simulink model "system"  (R2024b)
settings: Solver=FixedStepDiscrete  StartTime=0.0  StopTime=10.0  RelTol=1e-3
model workspace (MAT data in the model file):
  Risks = Simulink.Bus
  Risks.Alignment = -1
  Risks.PreserveElementDimensions = 0
  Risks.Elements_internal(1) = Simulink.BusElement
  Risks.Elements_internal(1).DimensionsMode = 'Fixed'
  Risks.Elements_internal(1).SamplingMode = 'Sample based'
  Risks.Elements_internal(1).SampleTime = -1
  Risks.Elements_internal(1).Name = 'VaR'
  Risks.Elements_internal(1).DataType_internal = 'double'
  Risks.Elements_internal(1).Complexity = 'real'
  Risks.Elements_internal(1).Dimensions = 1
  Risks.Elements_internal(2) = Simulink.BusElement
  Risks.Elements_internal(2).DimensionsMode = 'Fixed'
  Risks.Elements_internal(2).SamplingMode = 'Sample based'
  Risks.Elements_internal(2).SampleTime = -1
  Risks.Elements_internal(2).Name = 'liquidity'
  Risks.Elements_internal(2).DataType_internal = 'double'
  Risks.Elements_internal(2).Complexity = 'real'
  Risks.Elements_internal(2).Dimensions = 1
  Risks.Elements_internal(3) = Simulink.BusElement
  Risks.Elements_internal(3).DimensionsMode = 'Fixed'
  Risks.Elements_internal(3).SamplingMode = 'Sample based'
  Risks.Elements_internal(3).SampleTime = -1
  Risks.Elements_internal(3).Name = 'correlation'
  Risks.Elements_internal(3).DataType_internal = 'double'
  Risks.Elements_internal(3).Complexity = 'real'
  Risks.Elements_internal(3).Dimensions = 1
  Risks.Elements_internal(4) = Simulink.BusElement
  Risks.Elements_internal(4).DimensionsMode = 'Fixed'
  Risks.Elements_internal(4).SamplingMode = 'Sample based'
  Risks.Elements_internal(4).SampleTime = -1
  Risks.Elements_internal(4).Name = 'wavelet_coherence'
  Risks.Elements_internal(4).DataType_internal = 'double'
  Risks.Elements_internal(4).Complexity = 'real'
  Risks.Elements_internal(4).Dimensions = 1
  Risks.Elements_internal(5) = Simulink.BusElement
  Risks.Elements_internal(5).DimensionsMode = 'Fixed'
  Risks.Elements_internal(5).SamplingMode = 'Sample based'
  Risks.Elements_internal(5).SampleTime = -1
  Risks.Elements_internal(5).Name = 'crossMFDFA'
  Risks.Elements_internal(5).DataType_internal = 'double'
  Risks.Elements_internal(5).Complexity = 'real'
  Risks.Elements_internal(5).Dimensions = 1
  Risks.DataScope = 'Auto'
undefined symbols (not defined in the file): AA, Risk, UI
settings Model: Creator=lenskiy  LastModifiedBy=nagi
settings OptimizationCC: EnhancedBackFolding=on  PassReuseOutputArgsThreshold=0  ZeroExternalMemoryAtStartup=off  ZeroInternalMemoryAtStartup=off  MaxStackSize=64  OptimizeBlockOrder=speed  DifferentSizesBufferReuse=on  OptimizationCustomize=off
settings DebuggingCC: ParameterTunabilityLossMsg=error
settings HardwareCC: ProdBitPerLong=64  ProdHWDeviceType=Intel->x86-64 (MAC OS X)  UseEmbeddedCoderFeatures=off
settings SFSimCC: MATLABDynamicMemAlloc=off
settings RTWCC: Description=Embedded Coder  SystemTargetFile=ert.tlc  HardwareBoard=Robot Operating System 2 (ROS 2)  TLCOptions="-aInlineSetEventsForThisBaseRateFcn=TLC_FALSE -aSuppressMultiTaskScheduler=TLC_FALSE  -aRateBasedStepFcn=0"  TemplateMakefile=ert_default_tmf  Toolchain=Colcon Tools  TargetLang=C++
settings CodeAppCC: ForceParamTrailComments=on  OperatorAnnotations=on
settings ERTTargetCC: ERTCustomFileBanners=off  CodeInterfacePackaging=C++ class  SupportContinuousTime=on  SupportNonInlinedSFcns=on  RemoveResetFunc=off  ModelStepFunctionPrototypeControlCompliant=off  InlinedParameterPlacement=Hierarchical  RootIOFormat=Structure reference  DynamicArrayContainerType=coder::array

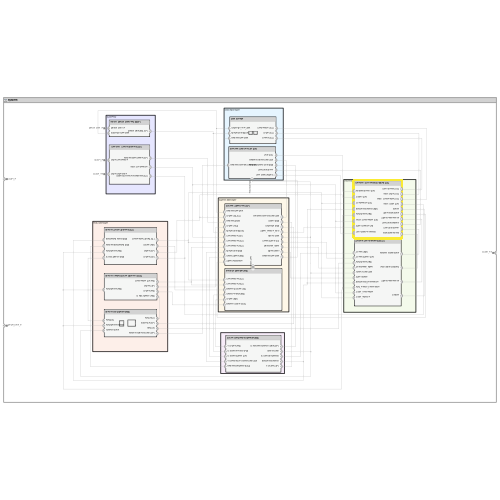
[thumbnail: Simulink's stored preview of the top-level diagram]
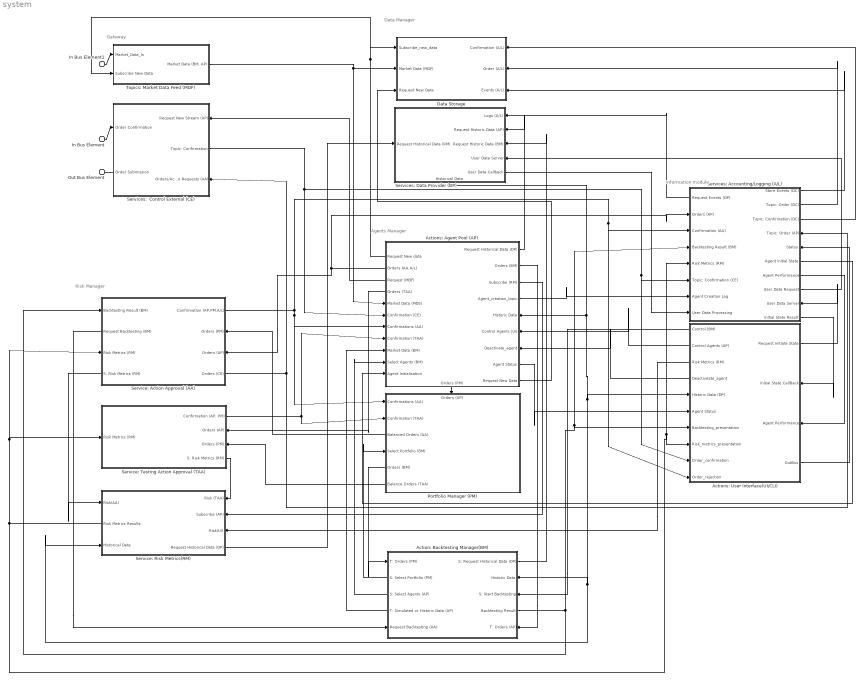
== system system ==
  note: Agents Manager
  note: Risk Manager
  note: Information module
  note: Data Manager
  note: Gateway
  In Bus Element : Inport  PortName=CCAPI_in
  In Bus Element1 : Inport  Port=2  PortName=Market_Data_In
  "  Services:  Control External (CE)" : Subsystem
      settings: PortSchema="{\"entries\":[{\"content\":{\"headerSize\":26,\"margin\":15,\"minimumSpacing\":25,\"sides\":[{\"content\":{\"connectorIds\":[\"In3\",\"Out1\"]},\"type\":\"ConnectorPlacement.EquallySpacedRectSide\",\"uuid\":\"c7e54eda-a439-456a-891f-e8c098e73b96\"},{\"content\":{\"connectorIds\":[\"In1\",\"Out2\",\"In2\"],\"side\":\"RIGHT\"},\"type\":\"ConnectorPlacement.EquallySpacedRectSide\",\"uuid\":\"93d01d87-f209-49b1-9fea-6a6e1e49cb0b\"},{\"content\":{\"side\":\"TOP\"},\"type\":\"ConnectorPlacement.EquallySpacedRectSide\",\"uuid\":\"f0abbd0b-06c8-4244-9bda-d971a55bccc5\"},{\"content\":{\"side\":\"BOTTOM\"},\"type\":\"ConnectorPlacement.EquallySpacedRectSide\",\"uuid\":\"d0091bd5-d57f-475a-8bc6-bc66948a1d1d\"}]},\"type\":\"ConnectorPlacement.EquallySpacedConnector\",\"uuid\":\"cf42f307-3a29-44ef-94e0-20f9bb6c1c81\"}],\"packageUris\":[\"http://schema.mathworks.com/mf0/Connector/R2020b\"],\"version\":\"1.0\"}"
  "Action: Backtesting Manager(BM) " : Subsystem
      settings: PortSchema="{\"entries\":[{\"content\":{\"headerSize\":26,\"margin\":15,\"minimumSpacing\":25,\"sides\":[{\"content\":{\"connectorIds\":[\"In4\",\"Out2\",\"Out4\",\"Out3\",\"In3\"]},\"type\":\"ConnectorPlacement.EquallySpacedRectSide\",\"uuid\":\"c7e54eda-a439-456a-891f-e8c098e73b96\"},{\"content\":{\"connectorIds\":[\"Out5\",\"In1\",\"In2\",\"Out1\",\"In5\"],\"side\":\"RIGHT\"},\"type\":\"ConnectorPlacement.EquallySpacedRectSide\",\"uuid\":\"93d01d87-f209-49b1-9fea-6a6e1e49cb0b\"},{\"content\":{\"side\":\"TOP\"},\"type\":\"ConnectorPlacement.EquallySpacedRectSide\",\"uuid\":\"f0abbd0b-06c8-4244-9bda-d971a55bccc5\"},{\"content\":{\"side\":\"BOTTOM\"},\"type\":\"ConnectorPlacement.EquallySpacedRectSide\",\"uuid\":\"c7ce6db1-31da-416d-9401-48a4b61b54ad\"}]},\"type\":\"ConnectorPlacement.EquallySpacedConnector\",\"uuid\":\"cf42f307-3a29-44ef-94e0-20f9bb6c1c81\"}],\"packageUris\":[\"http://schema.mathworks.com/mf0/Connector/R2020b\"],\"version\":\"1.0\"}"
  Actions: Agent Pool (AP) : Subsystem
      settings: PortSchema="{\"entries\":[{\"content\":{\"headerSize\":26,\"margin\":15,\"minimumSpacing\":25,\"sides\":[{\"content\":{\"connectorIds\":[\"Out8\",\"Out6\",\"Out5\",\"Out2\",\"In8\",\"In4\",\"In7\",\"In3\",\"In6\",\"In2\",\"In10\"]},\"type\":\"ConnectorPlacement.EquallySpacedRectSide\",\"uuid\":\"c7e54eda-a439-456a-891f-e8c098e73b96\"},{\"content\":{\"connectorIds\":[\"Out7\",\"Out3\",\"Out4\",\"Out10\",\"In1\",\"In5\",\"In9\",\"Out9\",\"Out11\"],\"side\":\"RIGHT\"},\"type\":\"ConnectorPlacement.EquallySpacedRectSide\",\"uuid\":\"93d01d87-f209-49b1-9fea-6a6e1e49cb0b\"},{\"content\":{\"side\":\"TOP\"},\"type\":\"ConnectorPlacement.EquallySpacedRectSide\",\"uuid\":\"f0abbd0b-06c8-4244-9bda-d971a55bccc5\"},{\"content\":{\"connectorIds\":[\"Out1\"],\"side\":\"BOTTOM\"},\"type\":\"ConnectorPlacement.EquallySpacedRectSide\",\"uuid\":\"897f63fa-91c4-4177-8500-44381925c77f\"}]},\"type\":\"ConnectorPlacement.EquallySpacedConnector\",\"uuid\":\"cf42f307-3a29-44ef-94e0-20f9bb6c1c81\"}],\"packageUris\":[\"http://schema.mathworks.com/mf0/Connector/R2020b\"],\"version\":\"1.0\"}"
  Actions: User Interface(UI/CLI) : Subsystem
      settings: PortSchema="{\"entries\":[{\"content\":{\"headerSize\":26,\"margin\":15,\"minimumSpacing\":25,\"sides\":[{\"content\":{\"connectorIds\":[\"Out3\",\"Out4\",\"Out2\",\"Out6\",\"In1\",\"In3\",\"In4\",\"In5\",\"In6\",\"In7\"]},\"type\":\"ConnectorPlacement.EquallySpacedRectSide\",\"uuid\":\"c7e54eda-a439-456a-891f-e8c098e73b96\"},{\"content\":{\"connectorIds\":[\"Out5\",\"In2\",\"In8\",\"Out1\"],\"side\":\"RIGHT\"},\"type\":\"ConnectorPlacement.EquallySpacedRectSide\",\"uuid\":\"93d01d87-f209-49b1-9fea-6a6e1e49cb0b\"},{\"content\":{\"side\":\"TOP\"},\"type\":\"ConnectorPlacement.EquallySpacedRectSide\",\"uuid\":\"f0abbd0b-06c8-4244-9bda-d971a55bccc5\"},{\"content\":{\"side\":\"BOTTOM\"},\"type\":\"ConnectorPlacement.EquallySpacedRectSide\",\"uuid\":\"239dc4b0-7955-4c14-b3b1-3030c8a0e9ad\"}]},\"type\":\"ConnectorPlacement.EquallySpacedConnector\",\"uuid\":\"cf42f307-3a29-44ef-94e0-20f9bb6c1c81\"}],\"packageUris\":[\"http://schema.mathworks.com/mf0/Connector/R2020b\"],\"version\":\"1.0\"}"
  Data Storage : Subsystem
      settings: PortSchema="{\"entries\":[{\"content\":{\"headerSize\":26,\"margin\":15,\"minimumSpacing\":25,\"sides\":[{\"content\":{\"connectorIds\":[\"In5\",\"In2\",\"In6\"]},\"type\":\"ConnectorPlacement.EquallySpacedRectSide\",\"uuid\":\"c7e54eda-a439-456a-891f-e8c098e73b96\"},{\"content\":{\"connectorIds\":[\"In3\",\"In4\",\"In1\"],\"side\":\"RIGHT\"},\"type\":\"ConnectorPlacement.EquallySpacedRectSide\",\"uuid\":\"93d01d87-f209-49b1-9fea-6a6e1e49cb0b\"},{\"content\":{\"side\":\"TOP\"},\"type\":\"ConnectorPlacement.EquallySpacedRectSide\",\"uuid\":\"f0abbd0b-06c8-4244-9bda-d971a55bccc5\"},{\"content\":{\"side\":\"BOTTOM\"},\"type\":\"ConnectorPlacement.EquallySpacedRectSide\",\"uuid\":\"d3fd7ded-18bf-4804-97b5-79887e5eea75\"}]},\"type\":\"ConnectorPlacement.EquallySpacedConnector\",\"uuid\":\"cf42f307-3a29-44ef-94e0-20f9bb6c1c81\"}],\"packageUris\":[\"http://schema.mathworks.com/mf0/Connector/R2020b\"],\"version\":\"1.0\"}"
  Portfolio Manager (PM) : Subsystem
      settings: PortSchema="{\"entries\":[{\"content\":{\"headerSize\":26,\"margin\":15,\"minimumSpacing\":25,\"sides\":[{\"content\":{\"connectorIds\":[\"In2\",\"In4\",\"Out3\",\"In1\",\"Out1\",\"Out2\"]},\"type\":\"ConnectorPlacement.EquallySpacedRectSide\",\"uuid\":\"c7e54eda-a439-456a-891f-e8c098e73b96\"},{\"content\":{\"side\":\"RIGHT\"},\"type\":\"ConnectorPlacement.EquallySpacedRectSide\",\"uuid\":\"93d01d87-f209-49b1-9fea-6a6e1e49cb0b\"},{\"content\":{\"connectorIds\":[\"In3\"],\"side\":\"TOP\"},\"type\":\"ConnectorPlacement.EquallySpacedRectSide\",\"uuid\":\"f0abbd0b-06c8-4244-9bda-d971a55bccc5\"},{\"content\":{\"side\":\"BOTTOM\"},\"type\":\"ConnectorPlacement.EquallySpacedRectSide\",\"uuid\":\"c17b4fb6-208b-4b15-8ab9-f7677697b6e9\"}]},\"type\":\"ConnectorPlacement.EquallySpacedConnector\",\"uuid\":\"cf42f307-3a29-44ef-94e0-20f9bb6c1c81\"}],\"packageUris\":[\"http://schema.mathworks.com/mf0/Connector/R2020b\"],\"version\":\"1.0\"}"
  Service: Action Approval (AA) : Subsystem
      settings: PortSchema="{\"entries\":[{\"content\":{\"headerSize\":26,\"margin\":15,\"minimumSpacing\":25,\"sides\":[{\"content\":{\"connectorIds\":[\"In1\",\"Out4\",\"In4\",\"Out1\"]},\"type\":\"ConnectorPlacement.EquallySpacedRectSide\",\"uuid\":\"c7e54eda-a439-456a-891f-e8c098e73b96\"},{\"content\":{\"connectorIds\":[\"Out3\",\"In2\",\"In3\",\"Out2\"],\"side\":\"RIGHT\"},\"type\":\"ConnectorPlacement.EquallySpacedRectSide\",\"uuid\":\"93d01d87-f209-49b1-9fea-6a6e1e49cb0b\"},{\"content\":{\"side\":\"TOP\"},\"type\":\"ConnectorPlacement.EquallySpacedRectSide\",\"uuid\":\"f0abbd0b-06c8-4244-9bda-d971a55bccc5\"},{\"content\":{\"side\":\"BOTTOM\"},\"type\":\"ConnectorPlacement.EquallySpacedRectSide\",\"uuid\":\"404a1439-590f-4a61-8168-47d1c9a050f4\"}]},\"type\":\"ConnectorPlacement.EquallySpacedConnector\",\"uuid\":\"cf42f307-3a29-44ef-94e0-20f9bb6c1c81\"}],\"packageUris\":[\"http://schema.mathworks.com/mf0/Connector/R2020b\"],\"version\":\"1.0\"}"
  Service: Risk Metrics(RM) : Subsystem
      settings: PortSchema="{\"entries\":[{\"content\":{\"headerSize\":26,\"margin\":15,\"minimumSpacing\":25,\"sides\":[{\"content\":{\"connectorIds\":[\"In3\",\"Out1\",\"In5\"]},\"type\":\"ConnectorPlacement.EquallySpacedRectSide\",\"uuid\":\"c7e54eda-a439-456a-891f-e8c098e73b96\"},{\"content\":{\"connectorIds\":[\"In1\",\"In4\",\"In2\",\"Out2\"],\"side\":\"RIGHT\"},\"type\":\"ConnectorPlacement.EquallySpacedRectSide\",\"uuid\":\"93d01d87-f209-49b1-9fea-6a6e1e49cb0b\"},{\"content\":{\"side\":\"TOP\"},\"type\":\"ConnectorPlacement.EquallySpacedRectSide\",\"uuid\":\"f0abbd0b-06c8-4244-9bda-d971a55bccc5\"},{\"content\":{\"side\":\"BOTTOM\"},\"type\":\"ConnectorPlacement.EquallySpacedRectSide\",\"uuid\":\"1a2f452a-f007-439c-b229-615c9b87871c\"}]},\"type\":\"ConnectorPlacement.EquallySpacedConnector\",\"uuid\":\"cf42f307-3a29-44ef-94e0-20f9bb6c1c81\"}],\"packageUris\":[\"http://schema.mathworks.com/mf0/Connector/R2020b\"],\"version\":\"1.0\"}"
  Service: Testing Action Approval (TAA) : Subsystem
      settings: PortSchema="{\"entries\":[{\"content\":{\"headerSize\":26,\"margin\":15,\"minimumSpacing\":25,\"sides\":[{\"content\":{\"connectorIds\":[\"In3\"]},\"type\":\"ConnectorPlacement.EquallySpacedRectSide\",\"uuid\":\"c7e54eda-a439-456a-891f-e8c098e73b96\"},{\"content\":{\"connectorIds\":[\"Out2\",\"In2\",\"In1\",\"Out1\"],\"side\":\"RIGHT\"},\"type\":\"ConnectorPlacement.EquallySpacedRectSide\",\"uuid\":\"93d01d87-f209-49b1-9fea-6a6e1e49cb0b\"},{\"content\":{\"side\":\"TOP\"},\"type\":\"ConnectorPlacement.EquallySpacedRectSide\",\"uuid\":\"f0abbd0b-06c8-4244-9bda-d971a55bccc5\"},{\"content\":{\"side\":\"BOTTOM\"},\"type\":\"ConnectorPlacement.EquallySpacedRectSide\",\"uuid\":\"404a1439-590f-4a61-8168-47d1c9a050f4\"}]},\"type\":\"ConnectorPlacement.EquallySpacedConnector\",\"uuid\":\"cf42f307-3a29-44ef-94e0-20f9bb6c1c81\"}],\"packageUris\":[\"http://schema.mathworks.com/mf0/Connector/R2020b\"],\"version\":\"1.0\"}"
  Services: Accounting/Logging (A/L) : Subsystem
      settings: PortSchema="{\"entries\":[{\"content\":{\"headerSize\":26,\"margin\":15,\"minimumSpacing\":25,\"sides\":[{\"content\":{\"connectorIds\":[\"Out1\",\"In1\",\"In2\",\"In6\",\"In7\",\"In4\",\"In8\",\"In9\"]},\"type\":\"ConnectorPlacement.EquallySpacedRectSide\",\"uuid\":\"c7e54eda-a439-456a-891f-e8c098e73b96\"},{\"content\":{\"connectorIds\":[\"Out2\",\"Out4\",\"Out3\",\"In5\",\"In3\",\"Out5\",\"Out6\",\"Out7\",\"In10\",\"Out8\"],\"side\":\"RIGHT\"},\"type\":\"ConnectorPlacement.EquallySpacedRectSide\",\"uuid\":\"93d01d87-f209-49b1-9fea-6a6e1e49cb0b\"},{\"content\":{\"side\":\"TOP\"},\"type\":\"ConnectorPlacement.EquallySpacedRectSide\",\"uuid\":\"f0abbd0b-06c8-4244-9bda-d971a55bccc5\"},{\"content\":{\"side\":\"BOTTOM\"},\"type\":\"ConnectorPlacement.EquallySpacedRectSide\",\"uuid\":\"8932d7e1-f270-4d28-9443-134a4dd6acae\"}]},\"type\":\"ConnectorPlacement.EquallySpacedConnector\",\"uuid\":\"cf42f307-3a29-44ef-94e0-20f9bb6c1c81\"}],\"packageUris\":[\"http://schema.mathworks.com/mf0/Connector/R2020b\"],\"version\":\"1.0\"}"
  Services: Data Provider (DP) : Subsystem
      settings: PortSchema="{\"entries\":[{\"content\":{\"headerSize\":26,\"margin\":15,\"minimumSpacing\":25,\"sides\":[{\"content\":{\"connectorIds\":[\"In4\"]},\"type\":\"ConnectorPlacement.EquallySpacedRectSide\",\"uuid\":\"c7e54eda-a439-456a-891f-e8c098e73b96\"},{\"content\":{\"connectorIds\":[\"In1\",\"In3\",\"In2\",\"In5\",\"Out2\"],\"side\":\"RIGHT\"},\"type\":\"ConnectorPlacement.EquallySpacedRectSide\",\"uuid\":\"93d01d87-f209-49b1-9fea-6a6e1e49cb0b\"},{\"content\":{\"side\":\"TOP\"},\"type\":\"ConnectorPlacement.EquallySpacedRectSide\",\"uuid\":\"f0abbd0b-06c8-4244-9bda-d971a55bccc5\"},{\"content\":{\"connectorIds\":[\"Out1\"],\"side\":\"BOTTOM\"},\"type\":\"ConnectorPlacement.EquallySpacedRectSide\",\"uuid\":\"d3fd7ded-18bf-4804-97b5-79887e5eea75\"}]},\"type\":\"ConnectorPlacement.EquallySpacedConnector\",\"uuid\":\"cf42f307-3a29-44ef-94e0-20f9bb6c1c81\"}],\"packageUris\":[\"http://schema.mathworks.com/mf0/Connector/R2020b\"],\"version\":\"1.0\"}"
  Topics: Market Data Feed (MDF) : Subsystem
      settings: PortSchema="{\"entries\":[{\"content\":{\"headerSize\":26,\"margin\":15,\"minimumSpacing\":25,\"sides\":[{\"content\":{\"connectorIds\":[\"In1\",\"In2\"]},\"type\":\"ConnectorPlacement.EquallySpacedRectSide\",\"uuid\":\"c7e54eda-a439-456a-891f-e8c098e73b96\"},{\"content\":{\"connectorIds\":[\"Out1\"],\"side\":\"RIGHT\"},\"type\":\"ConnectorPlacement.EquallySpacedRectSide\",\"uuid\":\"93d01d87-f209-49b1-9fea-6a6e1e49cb0b\"},{\"content\":{\"side\":\"TOP\"},\"type\":\"ConnectorPlacement.EquallySpacedRectSide\",\"uuid\":\"f0abbd0b-06c8-4244-9bda-d971a55bccc5\"},{\"content\":{\"side\":\"BOTTOM\"},\"type\":\"ConnectorPlacement.EquallySpacedRectSide\",\"uuid\":\"d0091bd5-d57f-475a-8bc6-bc66948a1d1d\"}]},\"type\":\"ConnectorPlacement.EquallySpacedConnector\",\"uuid\":\"cf42f307-3a29-44ef-94e0-20f9bb6c1c81\"}],\"packageUris\":[\"http://schema.mathworks.com/mf0/Connector/R2020b\"],\"version\":\"1.0\"}"
  Out Bus Element : Outport  PortName=CCAPI_out
  wires:
  Topics: Market Data Feed (MDF)/1("Market Data (BM, AP)") -> Actions: Agent Pool (AP)/8(Market Data (MDS)), Data Storage/2(Market Data (MDF))
  Actions: Agent Pool (AP)/6(Orders (AA,A/L)) -> Service: Action Approval (AA)/3(Orders (AP)), Services: Accounting/Logging (A/L)/1(Orders (AP))
  Service: Action Approval (AA)/3(Confirmation (AP,PM,A/L)) -> Actions: User Interface(UI/CLI)/7(Order_rejection), Services: Accounting/Logging (A/L)/2(Confirmation (AA)), Portfolio Manager (PM)/2(Confirmations (AA)), Actions: Agent Pool (AP)/7(Confirmations (AA))
  Service: Action Approval (AA)/2(Orders (CE)) -> "  Services:  Control External (CE)"/2(Orders/Account Info Requests (AA)), Services: Accounting/Logging (A/L)/5(Topic: Order (AP))
  Service: Action Approval (AA)/1(S: Risk Metrics (RM)) -> Service: Risk Metrics(RM)/3(Risk(AA))
  Services: Data Provider (DP)/1(Historical Data) -> Service: Risk Metrics(RM)/5(Historical Data), "Action: Backtesting Manager(BM) "/1(Historic Data), Actions: User Interface(UI/CLI)/1(Historic Data (DP)), Actions: Agent Pool (AP)/1(Historic Data)
  Actions: User Interface(UI/CLI)/1(OutBus) -> Services: Accounting/Logging (A/L)/3(" Status")
  Actions: Agent Pool (AP)/5(Request (MDF)) -> "  Services:  Control External (CE)"/1(Request New Stream (AP))
  "Action: Backtesting Manager(BM) "/5(S: Request Historical Data (DP)) -> Services: Data Provider (DP)/2(Request Historic Data (BM))
  Services: Accounting/Logging (A/L)/2(Store Events (DC)) -> Data Storage/1(" Events (A/L)")
  "Action: Backtesting Manager(BM) "/4(S: Select Agents (AP)) -> Actions: Agent Pool (AP)/2(Select Agents (BM))
  "Action: Backtesting Manager(BM) "/3(T: Simulated or Historic Data (AP)) -> Actions: Agent Pool (AP)/6(Market Data (BM))
  Actions: Agent Pool (AP)/3(Orders (BM)) -> "Action: Backtesting Manager(BM) "/5(T: Orders (AP))
  Actions: User Interface(UI/CLI)/4(Control Agents (AP)) -> Actions: Agent Pool (AP)/5(Control Agents (UI))
  Actions: User Interface(UI/CLI)/3(Control (BM)) -> "Action: Backtesting Manager(BM) "/2(S: Start Backtesting)
  Actions: User Interface(UI/CLI)/2(Risk Metrics (RM)) -> Service: Risk Metrics(RM)/2(Risk(UI))
  Actions: Agent Pool (AP)/1(Orders (PM)) -> Portfolio Manager (PM)/3(Orders (AP))
  Portfolio Manager (PM)/3(Balanced Orders (AA)) -> Service: Action Approval (AA)/2(Orders (PM))
  Portfolio Manager (PM)/1(Orders (BM)) -> "Action: Backtesting Manager(BM) "/4(T: Orders (PM))
  "Action: Backtesting Manager(BM) "/2(S: Select Portfolio (PM)) -> Portfolio Manager (PM)/1(Select Portfolio (BM))
  Services: Accounting/Logging (A/L)/1(Request Events (DP)) -> Services: Data Provider (DP)/1(" Logs (A/L)")
  Actions: Agent Pool (AP)/2(Orders (TAA)) -> Service: Testing Action Approval (TAA)/2(Orders (AP))
  Service: Testing Action Approval (TAA)/2("Confirmation (AP, PM)") -> Actions: Agent Pool (AP)/3(Confirmation (TAA)), Portfolio Manager (PM)/4(Confirmation (TAA))
  Portfolio Manager (PM)/2(Balance Orders (TAA)) -> Service: Testing Action Approval (TAA)/1(Orders (PM))
  Service: Testing Action Approval (TAA)/1(S: Risk Metrics (RM)) -> Service: Risk Metrics(RM)/1(Risk (TAA))
  Service: Risk Metrics(RM)/1(Risk Metrics Results) -> Service: Action Approval (AA)/4(Risk Metrics (RM)), Service: Testing Action Approval (TAA)/3(Risk Metrics (RM)), Services: Accounting/Logging (A/L)/7(Risk Metrics (RM)), Actions: User Interface(UI/CLI)/5(Risk_metrics_presentation)
  Actions: Agent Pool (AP)/4(Subscribe (RM)) -> Service: Risk Metrics(RM)/4(Subscribe (AP))
  "  Services:  Control External (CE)"/1(Order Submission) -> Out Bus Element/1
  In Bus Element/1 -> "  Services:  Control External (CE)"/3(Order Confirmation)
  "  Services:  Control External (CE)"/2(Topic: Confirmation) -> Actions: Agent Pool (AP)/4(Confirmation (CE)), Actions: User Interface(UI/CLI)/6(Order_confirmation), Services: Accounting/Logging (A/L)/4(Topic: Confirmation (CE))
  Services: Accounting/Logging (A/L)/3(Topic: Confirmation (DC)) -> Data Storage/3(Confirmation (A/L))
  Services: Accounting/Logging (A/L)/4(Topic: Order (DC)) -> Data Storage/4(Order (A/L))
  In Bus Element1/1 -> Topics: Market Data Feed (MDF)/1(Market_Data_In)
  Service: Action Approval (AA)/4(Request Backtesting (BM)) -> "Action: Backtesting Manager(BM) "/3(Request Backtesting (AA))
  "Action: Backtesting Manager(BM) "/1(Backtesting Result) -> Services: Accounting/Logging (A/L)/6(Backtesting Result (BM)), Actions: User Interface(UI/CLI)/4(Backtesting_presentation), Service: Action Approval (AA)/1(Backtesting Result (BM))
  Actions: Agent Pool (AP)/7(Request Historical Data (DP)) -> Services: Data Provider (DP)/3(Request Historic Data (AP))
  Service: Risk Metrics(RM)/2(Request Historical Data (DP)) -> Services: Data Provider (DP)/4(Request Historical Data (RM))
  Actions: Agent Pool (AP)/8(Request New data) -> Topics: Market Data Feed (MDF)/2(Subscribe New Data), Data Storage/5(Subscribe_new_data)
  Services: Data Provider (DP)/2(User Data Callback) -> Services: Accounting/Logging (A/L)/9(User Data Processing)
  Actions: Agent Pool (AP)/9(Agent Status) -> Actions: User Interface(UI/CLI)/3(Agent Status)
  Actions: Agent Pool (AP)/10(Agent_creation_topic) -> Services: Accounting/Logging (A/L)/8(Agent Creation Log)
  Actions: User Interface(UI/CLI)/6(Deactiveate_agent) -> Actions: Agent Pool (AP)/9(Deactivate_agent)
  Actions: Agent Pool (AP)/11(Request New Data) -> Data Storage/6(Request New Data)
  Services: Accounting/Logging (A/L)/5(Agent Initial State) -> Actions: Agent Pool (AP)/10(Agent Initialisation)
  Services: Accounting/Logging (A/L)/6(Agent Performance) -> Actions: User Interface(UI/CLI)/8(Agent Performance)
  Services: Accounting/Logging (A/L)/7(User Data Request) -> Services: Data Provider (DP)/5(User Data Server)
  Actions: User Interface(UI/CLI)/5(Request Initiate State) -> Services: Accounting/Logging (A/L)/10(User Data Server)
  Services: Accounting/Logging (A/L)/8(Initial State Result) -> Actions: User Interface(UI/CLI)/2(Initial State CallBack)

== system system/  Services:  Control External (CE) ==
  Bus Element In2 : Inport  PortName=Request New Stream (AP)
  Bus Element In1 : Inport  Port=2  PortName=Orders/Account Info Requests (AA)
  Bus Element In3 : Inport  Port=3  PortName=Order Confirmation
  Bus Element Out3 : Outport  PortName=Order Submission
  Bus Element Out4 : Outport  Port=2  PortName=Topic: Confirmation

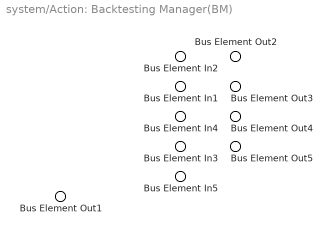
== system system/Action: Backtesting Manager(BM)  ==
  Bus Element In5 : Inport  PortName=Historic Data
  Bus Element In1 : Inport  Port=2  PortName=S: Start Backtesting
  Bus Element In3 : Inport  Port=3  PortName=Request Backtesting (AA)
  Bus Element In2 : Inport  Port=4  PortName=T: Orders (PM)
  Bus Element In4 : Inport  Port=5  PortName=T: Orders (AP)
  Bus Element Out4 : Outport  PortName=Backtesting Result
  Bus Element Out5 : Outport  Port=2  PortName=S: Select Portfolio (PM)
  Bus Element Out3 : Outport  Port=3  PortName=T: Simulated or Historic Data (AP)
  Bus Element Out2 : Outport  Port=4  PortName=S: Select Agents (AP)
  Bus Element Out1 : Outport  Port=5  PortName=S: Request Historical Data (DP)

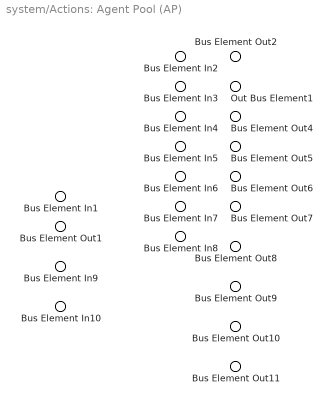
== system system/Actions: Agent Pool (AP) ==
  Bus Element In7 : Inport  PortName=Historic Data
  Bus Element In2 : Inport  Port=2  PortName=Select Agents (BM)
  Bus Element In6 : Inport  Port=3  PortName=Confirmation (TAA)
  Bus Element In8 : Inport  Port=4  PortName=Confirmation (CE)
  Bus Element In4 : Inport  Port=5  PortName=Control Agents (UI)
  Bus Element In5 : Inport  Port=6  PortName=Market Data (BM)
  Bus Element In3 : Inport  Port=7  PortName=Confirmations (AA)
  Bus Element In1 : Inport  Port=8  PortName=Market Data (MDS)
  Bus Element In9 : Inport  Port=9  PortName=Deactivate_agent
  Bus Element In10 : Inport  Port=10  PortName=Agent Initialisation
  Bus Element Out5 : Outport  PortName=Orders (PM)
  Bus Element Out6 : Outport  Port=2  PortName=Orders (TAA)
  Bus Element Out4 : Outport  Port=3  PortName=Orders (BM)
  Bus Element Out7 : Outport  Port=4  PortName=Subscribe (RM)
  Bus Element Out2 : Outport  Port=5  PortName=Request (MDF)
  Bus Element Out1 : Outport  Port=6  PortName=Orders (AA,A/L)
  Out Bus Element1 : Outport  Port=7  PortName=Request Historical Data (DP)
  Bus Element Out8 : Outport  Port=8  PortName=Request New data
  Bus Element Out9 : Outport  Port=9  PortName=Agent Status
  Bus Element Out10 : Outport  Port=10  PortName=Agent_creation_topic
  Bus Element Out11 : Outport  Port=11  PortName=Request New Data

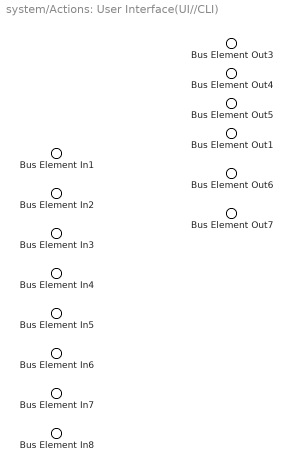
== system system/Actions: User Interface(UI//CLI) ==
  Bus Element In1 : Inport  PortName=Historic Data (DP)
  Bus Element In2 : Inport  Port=2  PortName=Initial State CallBack
  Bus Element In3 : Inport  Port=3  PortName=Agent Status
  Bus Element In4 : Inport  Port=4  PortName=Backtesting_presentation
  Bus Element In5 : Inport  Port=5  PortName=Risk_metrics_presentation
  Bus Element In6 : Inport  Port=6  PortName=Order_confirmation
  Bus Element In7 : Inport  Port=7  PortName=Order_rejection
  Bus Element In8 : Inport  Port=8  PortName=Agent Performance
  Bus Element Out1 : Outport  PortName=OutBus
  Bus Element Out5 : Outport  Port=2  PortName=Risk Metrics (RM)
  Bus Element Out4 : Outport  Port=3  PortName=Control (BM)
  Bus Element Out3 : Outport  Port=4  PortName=Control Agents (AP)
  Bus Element Out6 : Outport  Port=5  PortName=Request Initiate State
  Bus Element Out7 : Outport  Port=6  PortName=Deactiveate_agent

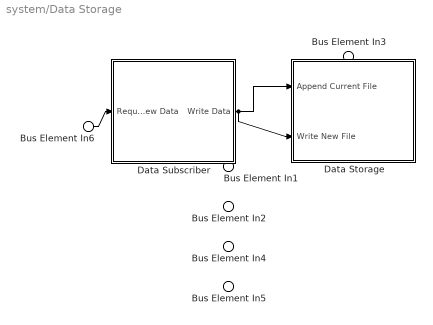
== system system/Data Storage ==
  Bus Element In3 : Inport  PortName=Events (A/L)
  Bus Element In1 : Inport  Port=2  PortName=Market Data (MDF)
  Bus Element In2 : Inport  Port=3  PortName=Confirmation (A/L)
  Bus Element In4 : Inport  Port=4  PortName=Order (A/L)
  Bus Element In5 : Inport  Port=5  PortName=Subscribe_new_data
  Bus Element In6 : Inport  Port=6  PortName=Request New Data
  Data Storage : Subsystem
      settings: PortSchema="{\"entries\":[{\"content\":{\"headerSize\":26,\"margin\":15,\"minimumSpacing\":25,\"sides\":[{\"content\":{\"connectorIds\":[\"In1\",\"In2\"]},\"type\":\"ConnectorPlacement.EquallySpacedRectSide\",\"uuid\":\"72b088da-6be2-4f39-86d9-1dec5d939a57\"},{\"content\":{\"side\":\"RIGHT\"},\"type\":\"ConnectorPlacement.EquallySpacedRectSide\",\"uuid\":\"3e630222-beed-4269-8eaa-e743757a473d\"},{\"content\":{\"side\":\"TOP\"},\"type\":\"ConnectorPlacement.EquallySpacedRectSide\",\"uuid\":\"e55fff88-3bcb-47c6-8712-517af8558fc3\"}]},\"type\":\"ConnectorPlacement.EquallySpacedConnector\",\"uuid\":\"d9b8126a-9f7a-4470-914d-1cf46528a28d\"}],\"packageUris\":[\"http://schema.mathworks.com/mf0/Connector/R2020b\"],\"version\":\"1.0\"}"
  Data Subscriber : Subsystem
      settings: PortSchema="{\"entries\":[{\"content\":{\"headerSize\":26,\"margin\":15,\"minimumSpacing\":25,\"sides\":[{\"content\":{\"connectorIds\":[\"In1\"]},\"type\":\"ConnectorPlacement.EquallySpacedRectSide\",\"uuid\":\"72b088da-6be2-4f39-86d9-1dec5d939a57\"},{\"content\":{\"connectorIds\":[\"Out1\"],\"side\":\"RIGHT\"},\"type\":\"ConnectorPlacement.EquallySpacedRectSide\",\"uuid\":\"3e630222-beed-4269-8eaa-e743757a473d\"},{\"content\":{\"side\":\"TOP\"},\"type\":\"ConnectorPlacement.EquallySpacedRectSide\",\"uuid\":\"e55fff88-3bcb-47c6-8712-517af8558fc3\"}]},\"type\":\"ConnectorPlacement.EquallySpacedConnector\",\"uuid\":\"d9b8126a-9f7a-4470-914d-1cf46528a28d\"}],\"packageUris\":[\"http://schema.mathworks.com/mf0/Connector/R2020b\"],\"version\":\"1.0\"}"
  wires:
  Data Subscriber/1(Write Data) -> Data Storage/2(Write New File), Data Storage/1(Append Current File)
  Bus Element In6/1 -> Data Subscriber/1(Request New Data)

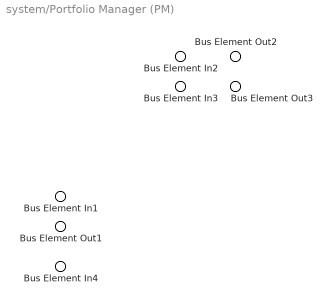
== system system/Portfolio Manager (PM) ==
  Bus Element In3 : Inport  PortName=Select Portfolio (BM)
  Bus Element In2 : Inport  Port=2  PortName=Confirmations (AA)
  Bus Element In1 : Inport  Port=3  PortName=Orders (AP)
  Bus Element In4 : Inport  Port=4  PortName=Confirmation (TAA)
  Bus Element Out2 : Outport  PortName=Orders (BM)
  Bus Element Out3 : Outport  Port=2  PortName=Balance Orders (TAA)
  Bus Element Out1 : Outport  Port=3  PortName=Balanced Orders (AA)

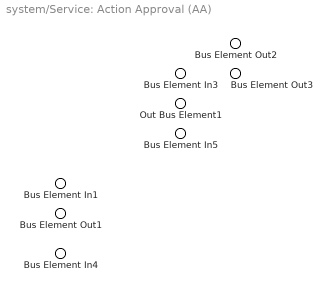
== system system/Service: Action Approval (AA) ==
  Bus Element In5 : Inport  PortName=Backtesting Result (BM)
  Bus Element In3 : Inport  Port=2  PortName=Orders (PM)
  Bus Element In1 : Inport  Port=3  PortName=Orders (AP)
  Bus Element In4 : Inport  Port=4  PortName=Risk Metrics (RM)
  Bus Element Out3 : Outport  PortName=S: Risk Metrics (RM)
  Bus Element Out2 : Outport  Port=2  PortName=Orders (CE)
  Bus Element Out1 : Outport  Port=3  PortName=Confirmation (AP,PM,A/L)
  Out Bus Element1 : Outport  Port=4  PortName=Request Backtesting (BM)

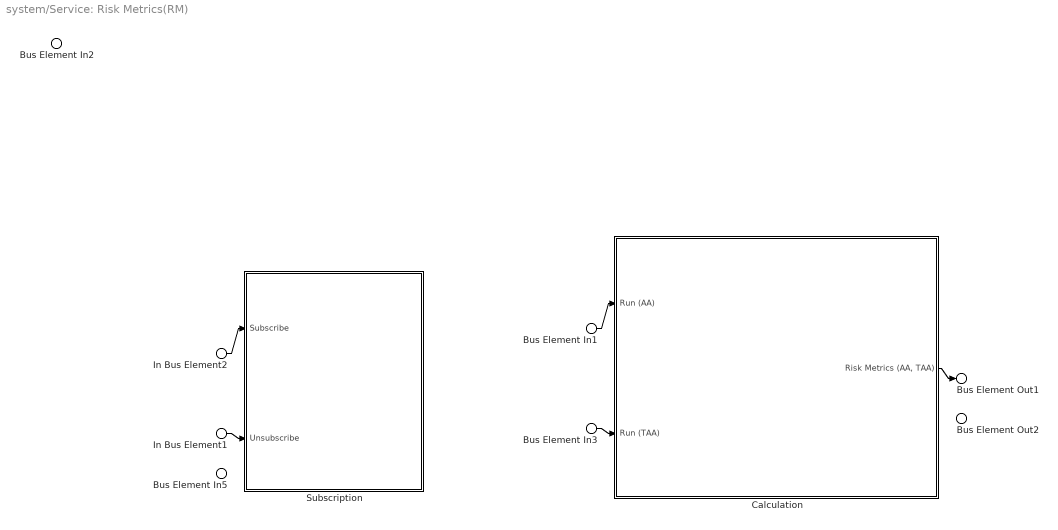
== system system/Service: Risk Metrics(RM) ==
  Bus Element In3 : Inport  PortName=Risk (TAA)
  Bus Element In2 : Inport  Port=2  PortName=Risk(UI)
  Bus Element In1 : Inport  Port=3  PortName=Risk(AA)
  In Bus Element2 : Inport  Port=4  PortName=Subscribe (AP)
  In Bus Element1 : Inport  Port=4  PortName=Subscribe (AP)
  Bus Element In5 : Inport  Port=5  PortName=Historical Data
  Calculation : Subsystem
      settings: PortSchema="{\"entries\":[{\"content\":{\"headerSize\":26,\"margin\":15,\"minimumSpacing\":25,\"sides\":[{\"content\":{\"connectorIds\":[\"In1\",\"In2\"]},\"type\":\"ConnectorPlacement.EquallySpacedRectSide\",\"uuid\":\"dd5ff5af-be48-4b61-a3ee-7d818d4cdc88\"},{\"content\":{\"connectorIds\":[\"Out1\"],\"side\":\"RIGHT\"},\"type\":\"ConnectorPlacement.EquallySpacedRectSide\",\"uuid\":\"02a6924d-a1b2-490b-997c-279faf232d36\"},{\"content\":{\"side\":\"TOP\"},\"type\":\"ConnectorPlacement.EquallySpacedRectSide\",\"uuid\":\"141c48b7-11a2-4087-8334-b2fd993d46dc\"}]},\"type\":\"ConnectorPlacement.EquallySpacedConnector\",\"uuid\":\"f405ae8c-72bf-4bdb-9e54-71737400ea90\"}],\"packageUris\":[\"http://schema.mathworks.com/mf0/Connector/R2020b\"],\"version\":\"1.0\"}"
  Subscription : Subsystem
      settings: PortSchema="{\"entries\":[{\"content\":{\"headerSize\":26,\"margin\":15,\"minimumSpacing\":25,\"sides\":[{\"content\":{\"connectorIds\":[\"In1\",\"In2\"]},\"type\":\"ConnectorPlacement.EquallySpacedRectSide\",\"uuid\":\"dd5ff5af-be48-4b61-a3ee-7d818d4cdc88\"},{\"content\":{\"side\":\"RIGHT\"},\"type\":\"ConnectorPlacement.EquallySpacedRectSide\",\"uuid\":\"02a6924d-a1b2-490b-997c-279faf232d36\"},{\"content\":{\"side\":\"TOP\"},\"type\":\"ConnectorPlacement.EquallySpacedRectSide\",\"uuid\":\"141c48b7-11a2-4087-8334-b2fd993d46dc\"}]},\"type\":\"ConnectorPlacement.EquallySpacedConnector\",\"uuid\":\"f405ae8c-72bf-4bdb-9e54-71737400ea90\"}],\"packageUris\":[\"http://schema.mathworks.com/mf0/Connector/R2020b\"],\"version\":\"1.0\"}"
  Bus Element Out1 : Outport  PortName=Risk Metrics Results
  Bus Element Out2 : Outport  Port=2  PortName=Request Historical Data (DP)
  wires:
  In Bus Element2/1 -> Subscription/1(Subscribe)
  In Bus Element1/1 -> Subscription/2(Unsubscribe)
  Bus Element In1/1 -> Calculation/1(Run (AA))
  Bus Element In3/1 -> Calculation/2(Run (TAA))
  Calculation/1("Risk Metrics (AA, TAA)") -> Bus Element Out1/1

== system system/Service: Testing Action Approval (TAA) ==
  Bus Element In3 : Inport  PortName=Orders (PM)
  Bus Element In1 : Inport  Port=2  PortName=Orders (AP)
  Bus Element In2 : Inport  Port=3  PortName=Risk Metrics (RM)
  Bus Element Out3 : Outport  PortName=S: Risk Metrics (RM)
  Bus Element Out1 : Outport  Port=2  PortName=Confirmation (AP, PM)

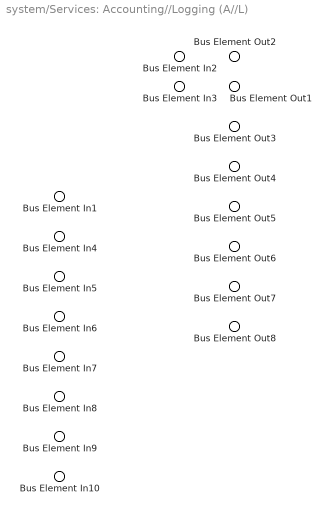
== system system/Services: Accounting//Logging (A//L) ==
  Bus Element In3 : Inport  PortName=Orders (AP)
  Bus Element In2 : Inport  Port=2  PortName=Confirmation (AA)
  Bus Element In1 : Inport  Port=3  PortName=Status
  Bus Element In4 : Inport  Port=4  PortName=Topic: Confirmation (CE)
  Bus Element In5 : Inport  Port=5  PortName=Topic: Order (AP)
  Bus Element In6 : Inport  Port=6  PortName=Backtesting Result (BM)
  Bus Element In7 : Inport  Port=7  PortName=Risk Metrics (RM)
  Bus Element In8 : Inport  Port=8  PortName=Agent Creation Log
  Bus Element In9 : Inport  Port=9  PortName=User Data Processing
  Bus Element In10 : Inport  Port=10  PortName=User Data Server
  Bus Element Out1 : Outport  PortName=Request Events (DP)
  Bus Element Out2 : Outport  Port=2  PortName=Store Events (DC)
  Bus Element Out3 : Outport  Port=3  PortName=Topic: Confirmation (DC)
  Bus Element Out4 : Outport  Port=4  PortName=Topic: Order (DC)
  Bus Element Out5 : Outport  Port=5  PortName=Agent Initial State
  Bus Element Out6 : Outport  Port=6  PortName=Agent Performance
  Bus Element Out7 : Outport  Port=7  PortName=User Data Request
  Bus Element Out8 : Outport  Port=8  PortName=Initial State Result

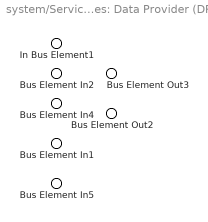
== system system/Services: Data Provider (DP) ==
  Bus Element In2 : Inport  PortName=Logs (A/L)
  Bus Element In4 : Inport  Port=2  PortName=Request Historic Data (BM)
  In Bus Element1 : Inport  Port=3  PortName=Request Historic Data (AP)
  Bus Element In1 : Inport  Port=4  PortName=Request Historical Data (RM)
  Bus Element In5 : Inport  Port=5  PortName=User Data Server
  Bus Element Out3 : Outport  PortName=Historical Data
  Bus Element Out2 : Outport  Port=2  PortName=User Data Callback

== system system/Topics: Market Data Feed (MDF) ==
  Bus Element In1 : Inport  PortName=Market_Data_In
  Bus Element In2 : Inport  Port=2  PortName=Subscribe New Data
  Bus Element Out1 : Outport  PortName=Market Data (BM, AP)

== system system/Data Storage/Data Storage ==
  Bus Element In1 : Inport  PortName=Append Current File
  Bus Element In2 : Inport  Port=2  PortName=Write New File

== system system/Data Storage/Data Subscriber ==
  Bus Element In1 : Inport  PortName=Request New Data
  Bus Element Out1 : Outport  PortName=Write Data

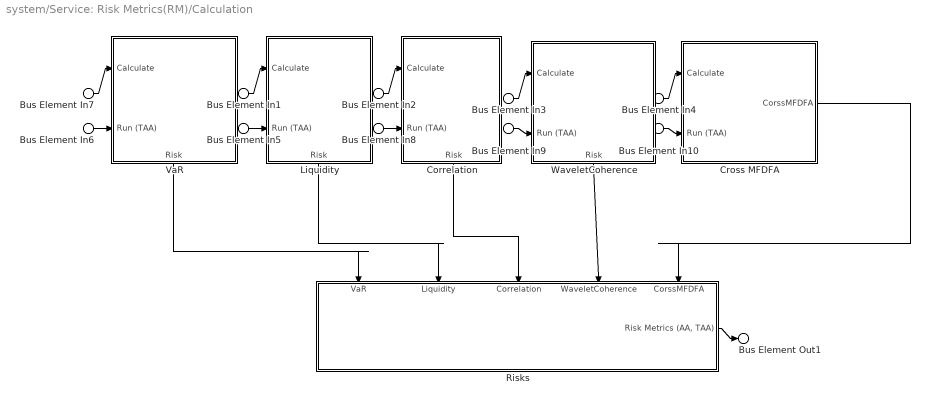
== system system/Service: Risk Metrics(RM)/Calculation ==
  Bus Element In{1..4,7} (5 alike) : Inport  PortName=Run (AA)
  Bus Element In{5..6,8..10} (5 alike) : Inport  Port=2  PortName=Run (TAA)
  Correlation : Subsystem
      settings: PortSchema="{\"entries\":[{\"content\":{\"headerSize\":26,\"margin\":15,\"minimumSpacing\":25,\"sides\":[{\"content\":{\"connectorIds\":[\"In1\",\"In2\"]},\"type\":\"ConnectorPlacement.EquallySpacedRectSide\",\"uuid\":\"dd5ff5af-be48-4b61-a3ee-7d818d4cdc88\"},{\"content\":{\"side\":\"RIGHT\"},\"type\":\"ConnectorPlacement.EquallySpacedRectSide\",\"uuid\":\"02a6924d-a1b2-490b-997c-279faf232d36\"},{\"content\":{\"side\":\"TOP\"},\"type\":\"ConnectorPlacement.EquallySpacedRectSide\",\"uuid\":\"141c48b7-11a2-4087-8334-b2fd993d46dc\"},{\"content\":{\"connectorIds\":[\"Out1\"],\"side\":\"BOTTOM\"},\"type\":\"ConnectorPlacement.EquallySpacedRectSide\",\"uuid\":\"c8d94622-5369-4926-ac8e-6b1b94c651e3\"}]},\"type\":\"ConnectorPlacement.EquallySpacedConnector\",\"uuid\":\"f405ae8c-72bf-4bdb-9e54-71737400ea90\"}],\"packageUris\":[\"http://schema.mathworks.com/mf0/Connector/R2020b\"],\"version\":\"1.0\"}"
  Cross MFDFA : Subsystem
      settings: PortSchema="{\"entries\":[{\"content\":{\"headerSize\":26,\"margin\":15,\"minimumSpacing\":25,\"sides\":[{\"content\":{\"connectorIds\":[\"In1\",\"In2\"]},\"type\":\"ConnectorPlacement.EquallySpacedRectSide\",\"uuid\":\"dd5ff5af-be48-4b61-a3ee-7d818d4cdc88\"},{\"content\":{\"connectorIds\":[\"Out1\"],\"side\":\"RIGHT\"},\"type\":\"ConnectorPlacement.EquallySpacedRectSide\",\"uuid\":\"02a6924d-a1b2-490b-997c-279faf232d36\"},{\"content\":{\"side\":\"TOP\"},\"type\":\"ConnectorPlacement.EquallySpacedRectSide\",\"uuid\":\"141c48b7-11a2-4087-8334-b2fd993d46dc\"},{\"content\":{\"side\":\"BOTTOM\"},\"type\":\"ConnectorPlacement.EquallySpacedRectSide\",\"uuid\":\"318bb783-36ea-4aa3-bd6c-38ef09b88506\"}]},\"type\":\"ConnectorPlacement.EquallySpacedConnector\",\"uuid\":\"f405ae8c-72bf-4bdb-9e54-71737400ea90\"}],\"packageUris\":[\"http://schema.mathworks.com/mf0/Connector/R2020b\"],\"version\":\"1.0\"}"
  Liquidity : Subsystem
      settings: PortSchema="{\"entries\":[{\"content\":{\"headerSize\":26,\"margin\":15,\"minimumSpacing\":25,\"sides\":[{\"content\":{\"connectorIds\":[\"In1\",\"In2\"]},\"type\":\"ConnectorPlacement.EquallySpacedRectSide\",\"uuid\":\"dd5ff5af-be48-4b61-a3ee-7d818d4cdc88\"},{\"content\":{\"side\":\"RIGHT\"},\"type\":\"ConnectorPlacement.EquallySpacedRectSide\",\"uuid\":\"02a6924d-a1b2-490b-997c-279faf232d36\"},{\"content\":{\"side\":\"TOP\"},\"type\":\"ConnectorPlacement.EquallySpacedRectSide\",\"uuid\":\"141c48b7-11a2-4087-8334-b2fd993d46dc\"},{\"content\":{\"connectorIds\":[\"Out1\"],\"side\":\"BOTTOM\"},\"type\":\"ConnectorPlacement.EquallySpacedRectSide\",\"uuid\":\"4fa86d91-e252-4fed-93db-0b64ea968a1f\"}]},\"type\":\"ConnectorPlacement.EquallySpacedConnector\",\"uuid\":\"f405ae8c-72bf-4bdb-9e54-71737400ea90\"}],\"packageUris\":[\"http://schema.mathworks.com/mf0/Connector/R2020b\"],\"version\":\"1.0\"}"
  Risks : Subsystem
      settings: PortSchema="{\"entries\":[{\"content\":{\"headerSize\":26,\"margin\":15,\"minimumSpacing\":25,\"sides\":[{\"content\":{},\"type\":\"ConnectorPlacement.EquallySpacedRectSide\",\"uuid\":\"dd5ff5af-be48-4b61-a3ee-7d818d4cdc88\"},{\"content\":{\"connectorIds\":[\"Out1\"],\"side\":\"RIGHT\"},\"type\":\"ConnectorPlacement.EquallySpacedRectSide\",\"uuid\":\"02a6924d-a1b2-490b-997c-279faf232d36\"},{\"content\":{\"connectorIds\":[\"In1\",\"In2\",\"In3\",\"In4\",\"In5\"],\"side\":\"TOP\"},\"type\":\"ConnectorPlacement.EquallySpacedRectSide\",\"uuid\":\"141c48b7-11a2-4087-8334-b2fd993d46dc\"}]},\"type\":\"ConnectorPlacement.EquallySpacedConnector\",\"uuid\":\"f405ae8c-72bf-4bdb-9e54-71737400ea90\"}],\"packageUris\":[\"http://schema.mathworks.com/mf0/Connector/R2020b\"],\"version\":\"1.0\"}"
  VaR : Subsystem
      settings: PortSchema="{\"entries\":[{\"content\":{\"headerSize\":26,\"margin\":15,\"minimumSpacing\":25,\"sides\":[{\"content\":{\"connectorIds\":[\"In1\",\"In2\"]},\"type\":\"ConnectorPlacement.EquallySpacedRectSide\",\"uuid\":\"dd5ff5af-be48-4b61-a3ee-7d818d4cdc88\"},{\"content\":{\"side\":\"RIGHT\"},\"type\":\"ConnectorPlacement.EquallySpacedRectSide\",\"uuid\":\"02a6924d-a1b2-490b-997c-279faf232d36\"},{\"content\":{\"side\":\"TOP\"},\"type\":\"ConnectorPlacement.EquallySpacedRectSide\",\"uuid\":\"141c48b7-11a2-4087-8334-b2fd993d46dc\"},{\"content\":{\"connectorIds\":[\"Out1\"],\"side\":\"BOTTOM\"},\"type\":\"ConnectorPlacement.EquallySpacedRectSide\",\"uuid\":\"b918c4be-b53c-43e3-b06e-d826fcfce314\"}]},\"type\":\"ConnectorPlacement.EquallySpacedConnector\",\"uuid\":\"f405ae8c-72bf-4bdb-9e54-71737400ea90\"}],\"packageUris\":[\"http://schema.mathworks.com/mf0/Connector/R2020b\"],\"version\":\"1.0\"}"
  WaveletCoherence : Subsystem
      settings: PortSchema="{\"entries\":[{\"content\":{\"headerSize\":26,\"margin\":15,\"minimumSpacing\":25,\"sides\":[{\"content\":{\"connectorIds\":[\"In1\",\"In2\"]},\"type\":\"ConnectorPlacement.EquallySpacedRectSide\",\"uuid\":\"dd5ff5af-be48-4b61-a3ee-7d818d4cdc88\"},{\"content\":{\"side\":\"RIGHT\"},\"type\":\"ConnectorPlacement.EquallySpacedRectSide\",\"uuid\":\"02a6924d-a1b2-490b-997c-279faf232d36\"},{\"content\":{\"side\":\"TOP\"},\"type\":\"ConnectorPlacement.EquallySpacedRectSide\",\"uuid\":\"141c48b7-11a2-4087-8334-b2fd993d46dc\"},{\"content\":{\"connectorIds\":[\"Out1\"],\"side\":\"BOTTOM\"},\"type\":\"ConnectorPlacement.EquallySpacedRectSide\",\"uuid\":\"4b4658a0-d0df-4ee1-b82c-ffc500e3ac80\"}]},\"type\":\"ConnectorPlacement.EquallySpacedConnector\",\"uuid\":\"f405ae8c-72bf-4bdb-9e54-71737400ea90\"}],\"packageUris\":[\"http://schema.mathworks.com/mf0/Connector/R2020b\"],\"version\":\"1.0\"}"
  Bus Element Out1 : Outport  PortName=Risk Metrics (AA, TAA)
  wires:
  Bus Element In7/1 -> VaR/1(Calculate)
  Bus Element In1/1 -> Liquidity/1(Calculate)
  Bus Element In2/1 -> Correlation/1(Calculate)
  Bus Element In3/1 -> WaveletCoherence/1(Calculate)
  Bus Element In4/1 -> Cross MFDFA/1(Calculate)
  Cross MFDFA/1(CorssMFDFA) -> Risks/5(CorssMFDFA)
  WaveletCoherence/1(Risk) -> Risks/4(WaveletCoherence)
  Correlation/1(Risk) -> Risks/3(Correlation)
  Liquidity/1(Risk) -> Risks/2(Liquidity)
  VaR/1(Risk) -> Risks/1(VaR)
  Risks/1("Risk Metrics (AA, TAA)") -> Bus Element Out1/1
  Bus Element In6/1 -> VaR/2(Run (TAA))
  Bus Element In5/1 -> Liquidity/2(Run (TAA))
  Bus Element In8/1 -> Correlation/2(Run (TAA))
  Bus Element In9/1 -> WaveletCoherence/2(Run (TAA))
  Bus Element In10/1 -> Cross MFDFA/2(Run (TAA))

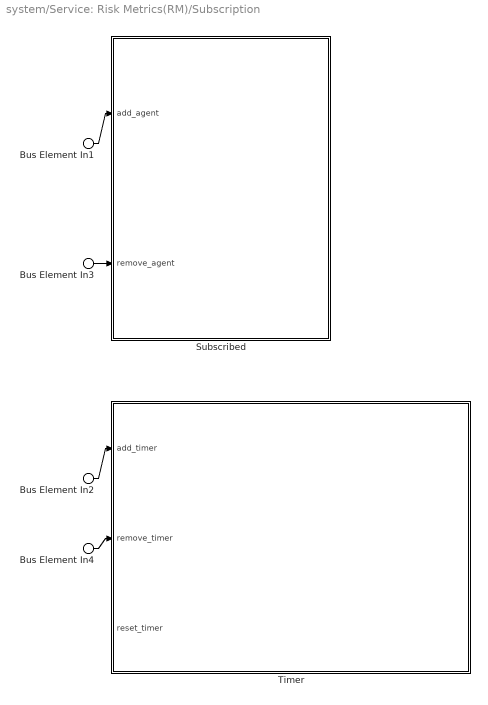
== system system/Service: Risk Metrics(RM)/Subscription ==
  Bus Element In1 : Inport  PortName=Subscribe
  Bus Element In2 : Inport  PortName=Subscribe
  Bus Element In3 : Inport  Port=2  PortName=Unsubscribe
  Bus Element In4 : Inport  Port=2  PortName=Unsubscribe
  Subscribed : Subsystem
      settings: PortSchema="{\"entries\":[{\"content\":{\"headerSize\":26,\"margin\":15,\"minimumSpacing\":25,\"sides\":[{\"content\":{\"connectorIds\":[\"In1\",\"In2\"]},\"type\":\"ConnectorPlacement.EquallySpacedRectSide\",\"uuid\":\"dd5ff5af-be48-4b61-a3ee-7d818d4cdc88\"},{\"content\":{\"side\":\"RIGHT\"},\"type\":\"ConnectorPlacement.EquallySpacedRectSide\",\"uuid\":\"02a6924d-a1b2-490b-997c-279faf232d36\"},{\"content\":{\"side\":\"TOP\"},\"type\":\"ConnectorPlacement.EquallySpacedRectSide\",\"uuid\":\"141c48b7-11a2-4087-8334-b2fd993d46dc\"}]},\"type\":\"ConnectorPlacement.EquallySpacedConnector\",\"uuid\":\"f405ae8c-72bf-4bdb-9e54-71737400ea90\"}],\"packageUris\":[\"http://schema.mathworks.com/mf0/Connector/R2020b\"],\"version\":\"1.0\"}"
  Timer : Subsystem
      settings: PortSchema="{\"entries\":[{\"content\":{\"headerSize\":26,\"margin\":15,\"minimumSpacing\":25,\"sides\":[{\"content\":{\"connectorIds\":[\"In1\",\"In2\",\"In3\"]},\"type\":\"ConnectorPlacement.EquallySpacedRectSide\",\"uuid\":\"dd5ff5af-be48-4b61-a3ee-7d818d4cdc88\"},{\"content\":{\"side\":\"RIGHT\"},\"type\":\"ConnectorPlacement.EquallySpacedRectSide\",\"uuid\":\"02a6924d-a1b2-490b-997c-279faf232d36\"},{\"content\":{\"side\":\"TOP\"},\"type\":\"ConnectorPlacement.EquallySpacedRectSide\",\"uuid\":\"141c48b7-11a2-4087-8334-b2fd993d46dc\"}]},\"type\":\"ConnectorPlacement.EquallySpacedConnector\",\"uuid\":\"f405ae8c-72bf-4bdb-9e54-71737400ea90\"}],\"packageUris\":[\"http://schema.mathworks.com/mf0/Connector/R2020b\"],\"version\":\"1.0\"}"
  wires:
  Bus Element In1/1 -> Subscribed/1(add_agent)
  Bus Element In2/1 -> Timer/1(add_timer)
  Bus Element In3/1 -> Subscribed/2(remove_agent)
  Bus Element In4/1 -> Timer/2(remove_timer)

== system system/Service: Risk Metrics(RM)/Calculation/Correlation ==
  In Bus Element1 : Inport  PortName=Calculate
  Bus Element In2 : Inport  Port=2  PortName=Run (TAA)
  Bus Element Out1 : Outport  PortName=Risk

== system system/Service: Risk Metrics(RM)/Calculation/Cross MFDFA ==
  In Bus Element1 : Inport  PortName=Calculate
  Bus Element In2 : Inport  Port=2  PortName=Run (TAA)
  Bus Element Out1 : Outport  PortName=CorssMFDFA

== system system/Service: Risk Metrics(RM)/Calculation/Liquidity ==
  In Bus Element1 : Inport  PortName=Calculate
  Bus Element In2 : Inport  Port=2  PortName=Run (TAA)
  Bus Element Out1 : Outport  PortName=Risk

== system system/Service: Risk Metrics(RM)/Calculation/Risks ==
  Bus Element In5 : Inport  PortName=VaR
  Bus Element In4 : Inport  Port=2  PortName=Liquidity
  Bus Element In3 : Inport  Port=3  PortName=Correlation
  Bus Element In2 : Inport  Port=4  PortName=WaveletCoherence
  Bus Element In1 : Inport  Port=5  PortName=CorssMFDFA
  Bus Element Out1 : Outport  PortName=Risk Metrics (AA, TAA)

== system system/Service: Risk Metrics(RM)/Calculation/VaR ==
  In Bus Element1 : Inport  PortName=Calculate
  Bus Element In2 : Inport  Port=2  PortName=Run (TAA)
  Out Bus Element1 : Outport  PortName=Risk

== system system/Service: Risk Metrics(RM)/Calculation/WaveletCoherence ==
  In Bus Element1 : Inport  PortName=Calculate
  Bus Element In2 : Inport  Port=2  PortName=Run (TAA)
  Bus Element Out1 : Outport  PortName=Risk

== system system/Service: Risk Metrics(RM)/Subscription/Subscribed ==
  Bus Element In1 : Inport  PortName=add_agent
  Bus Element In2 : Inport  Port=2  PortName=remove_agent

== system system/Service: Risk Metrics(RM)/Subscription/Timer ==
  Bus Element In1 : Inport  PortName=add_timer
  Bus Element In2 : Inport  Port=2  PortName=remove_timer
  Bus Element In3 : Inport  Port=3  PortName=reset_timer
